simulink model "linear_model2"  (R2016b)
settings: Solver=ode4  StartTime=0.0  StopTime=10  FixedStep=0.02  RelTol=1e-3
values from neighbouring files (symbols this model uses):
  A = [0 1 0 0 ... (first row only)    [testLinearPara2.m]    (also in testLinearPara_speed.m = [ A1 A2 0)
  B = [0;B1;0;B2]    [testLinearPara2.m]    (also in testLinearPara_speed.m = [B1;0;B2])
  C = eye(4)    [testLinearPara2.m]    (also in testLinearPara_speed.m = eye(3))
  D = [0;0;0;0]    [testLinearPara2.m]    (also in testLinearPara_speed.m = [0;0;0])
  K = place(A, B, poles)    [testLinearPara2.m]    (also in testLinearPara_speed.m)
  K_deg = K    [testLinearPara2.m]    (also in testLinearPara_speed.m)
  rho = [0.699955193506 142.002353827 -0.10553969689 -0.297054783039]    [parameters2.mat]
  sig = [9.55300470583 0.353221407523 -232.496192342 4.24767719412]    [parameters2.mat]
undefined symbols (not defined in the file or in its folder): K_lqr
settings Model: Creator=Ernie  LastModifiedBy=Ernie

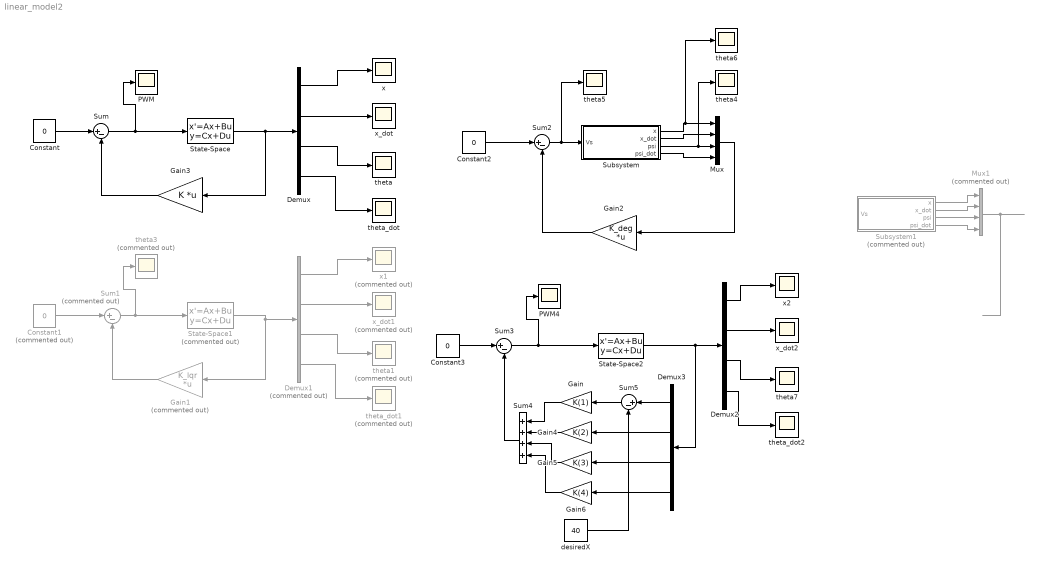
== system linear_model2 ==
  Constant : Constant  Value=0
  Constant1 : Constant  Commented=on  Value=0
  Constant2 : Constant  Value=0
  Constant3 : Constant  Value=0
  Demux : Demux
  Demux1 : Demux  Commented=on
  Demux2 : Demux
  Demux3 : Demux
  Gain : Gain  Gain=K(1)
  Gain1 : Gain  Commented=on  Gain=K_lqr  Multiplication=Matrix(K*u)
  Gain2 : Gain  Gain=K_deg  Multiplication=Matrix(K*u)
  Gain3 : Gain  Gain=K  Multiplication=Matrix(K*u)
  Gain4 : Gain  Gain=K(2)
  Gain5 : Gain  Gain=K(3)
  Gain6 : Gain  Gain=K(4)
  Mux : Mux
  Mux1 : Mux  Commented=on
  PWM : Scope
  PWM4 : Scope
  State-Space : StateSpace  A=A  B=B  C=C  D=D  X0=[0 0 0.1743 0]
  State-Space1 : StateSpace  Commented=on  A=A  B=B  C=C  D=D  X0=[ 0 0 0.1745 0]
  State-Space2 : StateSpace  A=A  B=B  C=C  D=D  X0=[0 0 0 0]
  Subsystem : Subsystem
  Subsystem1 : Subsystem  Commented=on
  Sum{,2..3,5} (4 alike) : Sum  Inputs=|+-
  Sum1 : Sum  Commented=on  Inputs=|+-
  Sum4 : Sum  Inputs=++++
  desiredX : Constant  Value=40
  theta{,4..7} (5 alike) : Scope
  theta1 : Scope  Commented=on
  theta3 : Scope  Commented=on
  theta_dot : Scope
  theta_dot1 : Scope  Commented=on
  theta_dot2 : Scope
  x : Scope
  x1 : Scope  Commented=on
  x2 : Scope
  x_dot : Scope
  x_dot1 : Scope  Commented=on
  x_dot2 : Scope
  wires:
  State-Space/1 -> Gain3/1, Demux/1
  Demux/1 -> x/1
  Demux/2 -> x_dot/1
  Demux/3 -> theta/1
  Demux/4 -> theta_dot/1
  State-Space1/1 -> Demux1/1, Gain1/1
  Gain1/1 -> Sum1/2
  Sum1/1 -> theta3/1, State-Space1/1
  Constant1/1 -> Sum1/1
  Demux1/1 -> x1/1
  Demux1/2 -> x_dot1/1
  Demux1/3 -> theta1/1
  Demux1/4 -> theta_dot1/1
  Subsystem/3(psi) -> theta4/1, Mux/3
  Subsystem/4(psi_dot) -> Mux/4
  Subsystem/1(x) -> theta6/1, Mux/1
  Subsystem/2(x_dot) -> Mux/2
  Mux/1 -> Gain2/1
  Gain2/1 -> Sum2/2
  Constant2/1 -> Sum2/1
  Sum2/1 -> theta5/1, Subsystem/1(Vs)
  Sum/1 -> State-Space/1, PWM/1
  Gain3/1 -> Sum/2
  Constant/1 -> Sum/1
  Demux2/1 -> x2/1
  Demux2/2 -> x_dot2/1
  Demux2/3 -> theta7/1
  Demux2/4 -> theta_dot2/1
  Constant3/1 -> Sum3/1
  Sum4/1 -> Sum3/2
  Gain/1 -> Sum4/1
  Gain4/1 -> Sum4/2
  Gain5/1 -> Sum4/3
  Gain6/1 -> Sum4/4
  Demux3/1 -> Sum5/1
  Sum5/1 -> Gain/1
  Demux3/3 -> Gain5/1
  Demux3/4 -> Gain6/1
  desiredX/1 -> Sum5/2
  Sum3/1 -> State-Space2/1, PWM4/1
  Mux1/1 -> ?
  ? -> Subsystem1/1(Vs)
  Subsystem1/3(psi) -> Mux1/3
  Subsystem1/4(psi_dot) -> Mux1/4
  Subsystem1/1(x) -> Mux1/1
  Subsystem1/2(x_dot) -> Mux1/2
  State-Space2/1 -> Demux3/1, Demux2/1
  Demux3/2 -> Gain4/1

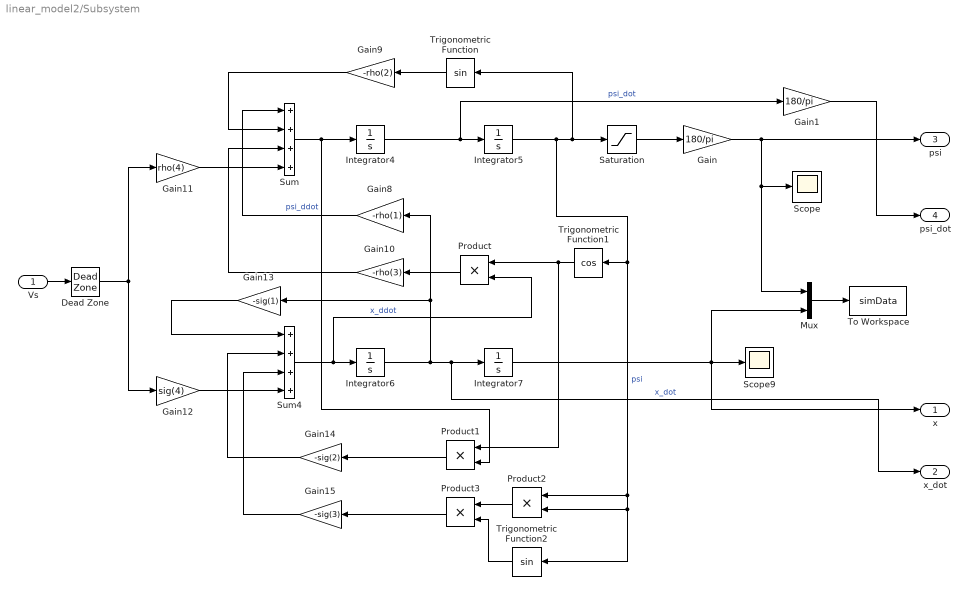
== system linear_model2/Subsystem ==
  Vs : Inport
  Dead Zone : DeadZone  LowerValue=-10  UpperValue=10  SaturateOnIntegerOverflow=on
  Gain : Gain  Gain=180/pi
  Gain1 : Gain  Gain=180/pi
  Gain10 : Gain  Gain=-rho(3)
  Gain11 : Gain  Gain=rho(4)
  Gain12 : Gain  Gain=sig(4)
  Gain13 : Gain  Gain=-sig(1)
  Gain14 : Gain  Gain=-sig(2)
  Gain15 : Gain  Gain=-sig(3)
  Gain8 : Gain  Gain=-rho(1)
  Gain9 : Gain  Gain=-rho(2)
  Integrator4 : Integrator
  Integrator5 : Integrator  InitialCondition=20*pi/180
  Integrator6 : Integrator
  Integrator7 : Integrator
  Mux : Mux  Inputs=2
  Product{,1..3} (4 alike) : Product
  Saturation : Saturate  UpperLimit=pi/2  LowerLimit=-pi/2
  Scope : Scope
  Scope9 : Scope
  Sum : Sum  Inputs=++++
  Sum4 : Sum  Inputs=++++
  To Workspace : ToWorkspace  VariableName=simData  SaveFormat=Timeseries  SampleTime=-1
  Trigonometric Function : Trigonometry
  Trigonometric Function1 : Trigonometry  Operator=cos
  Trigonometric Function2 : Trigonometry
  x : Outport
  x_dot : Outport  Port=2
  psi : Outport  Port=3
  psi_dot : Outport  Port=4
  wires:
  Integrator4/1 -> Gain1/1, Integrator5/1  "psi_dot"
  Integrator6/1 -> Gain13/1, Gain8/1, x_dot/1, Integrator7/1  "x_dot"
  Sum4/1 -> Product/2, Integrator6/1  "x_ddot"
  Sum/1 -> Product1/2, Integrator4/1  "psi_ddot"
  Gain8/1 -> Sum/1
  Trigonometric Function/1 -> Gain9/1
  Integrator5/1 -> Trigonometric Function2/1, Product2/2, Product2/1, Trigonometric Function1/1, Saturation/1, Trigonometric Function/1  "psi"
  Gain9/1 -> Sum/2
  Product/1 -> Gain10/1
  Trigonometric Function1/1 -> Product1/1, Product/1
  Gain10/1 -> Sum/3
  Gain11/1 -> Sum/4
  Gain12/1 -> Sum4/4
  Gain13/1 -> Sum4/1
  Product1/1 -> Gain14/1
  Gain14/1 -> Sum4/2
  Product2/1 -> Product3/1
  Trigonometric Function2/1 -> Product3/2
  Product3/1 -> Gain15/1
  Gain15/1 -> Sum4/3
  Integrator7/1 -> x/1, Mux/2, Scope9/1
  Mux/1 -> To Workspace/1
  Gain/1 -> Mux/1, Scope/1, psi/1
  Saturation/1 -> Gain/1
  Vs/1 -> Dead Zone/1
  Dead Zone/1 -> Gain12/1, Gain11/1
  Gain1/1 -> psi_dot/1

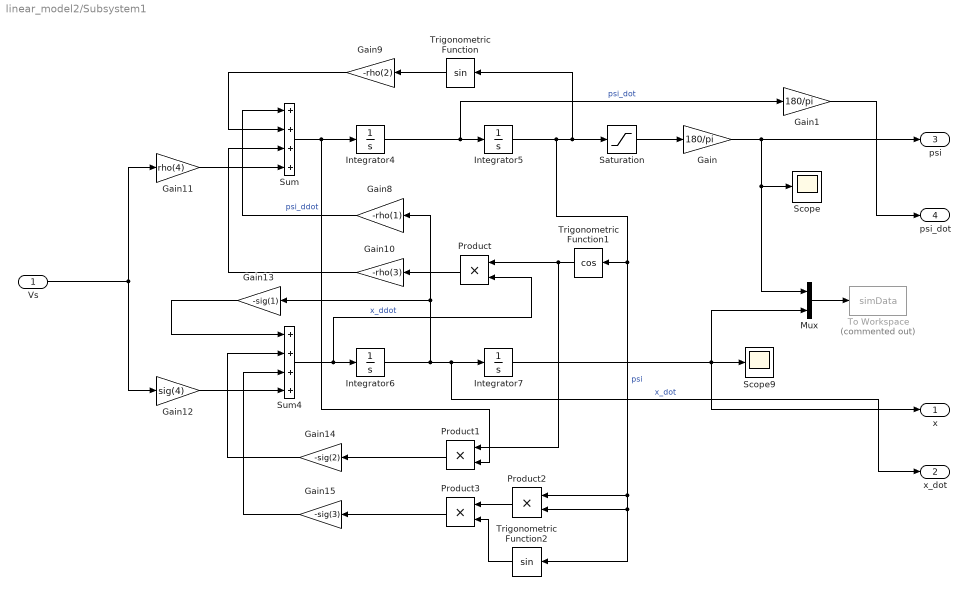
== system linear_model2/Subsystem1 ==
  Vs : Inport
  Gain : Gain  Gain=180/pi
  Gain1 : Gain  Gain=180/pi
  Gain10 : Gain  Gain=-rho(3)
  Gain11 : Gain  Gain=rho(4)
  Gain12 : Gain  Gain=sig(4)
  Gain13 : Gain  Gain=-sig(1)
  Gain14 : Gain  Gain=-sig(2)
  Gain15 : Gain  Gain=-sig(3)
  Gain8 : Gain  Gain=-rho(1)
  Gain9 : Gain  Gain=-rho(2)
  Integrator4 : Integrator
  Integrator5 : Integrator  InitialCondition=20*pi/180
  Integrator6 : Integrator
  Integrator7 : Integrator
  Mux : Mux  Inputs=2
  Product{,1..3} (4 alike) : Product
  Saturation : Saturate  UpperLimit=pi/2  LowerLimit=-pi/2
  Scope : Scope
  Scope9 : Scope
  Sum : Sum  Inputs=++++
  Sum4 : Sum  Inputs=++++
  To Workspace : ToWorkspace  Commented=on  VariableName=simData  SaveFormat=Timeseries  SampleTime=-1
  Trigonometric Function : Trigonometry
  Trigonometric Function1 : Trigonometry  Operator=cos
  Trigonometric Function2 : Trigonometry
  x : Outport
  x_dot : Outport  Port=2
  psi : Outport  Port=3
  psi_dot : Outport  Port=4
  wires:
  Integrator4/1 -> Gain1/1, Integrator5/1  "psi_dot"
  Integrator6/1 -> Gain13/1, Gain8/1, x_dot/1, Integrator7/1  "x_dot"
  Sum4/1 -> Product/2, Integrator6/1  "x_ddot"
  Sum/1 -> Product1/2, Integrator4/1  "psi_ddot"
  Gain8/1 -> Sum/1
  Trigonometric Function/1 -> Gain9/1
  Integrator5/1 -> Trigonometric Function2/1, Product2/2, Product2/1, Trigonometric Function1/1, Saturation/1, Trigonometric Function/1  "psi"
  Gain9/1 -> Sum/2
  Product/1 -> Gain10/1
  Trigonometric Function1/1 -> Product1/1, Product/1
  Gain10/1 -> Sum/3
  Gain11/1 -> Sum/4
  Gain12/1 -> Sum4/4
  Gain13/1 -> Sum4/1
  Product1/1 -> Gain14/1
  Gain14/1 -> Sum4/2
  Product2/1 -> Product3/1
  Trigonometric Function2/1 -> Product3/2
  Product3/1 -> Gain15/1
  Gain15/1 -> Sum4/3
  Integrator7/1 -> x/1, Mux/2, Scope9/1
  Mux/1 -> To Workspace/1
  Gain/1 -> Mux/1, Scope/1, psi/1
  Saturation/1 -> Gain/1
  Vs/1 -> Gain12/1, Gain11/1
  Gain1/1 -> psi_dot/1
